simulink library "RobotX_Lib"  (R2026a)
settings: Solver=VariableStepAuto
settings Model: Creator=shueb  LastModifiedBy=shueb

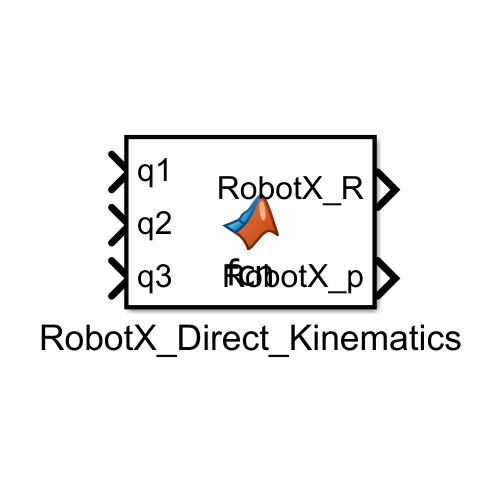
[thumbnail: Simulink's stored preview of the top-level diagram]
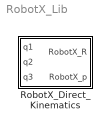
== system RobotX_Lib ==
  RobotX_Direct_Kinematics : MATLAB Function  TreatAsAtomicUnit=on

== matlab function RobotX_Lib/RobotX_Direct_Kinematics ==
  data: q1 input; RobotX_R output; q2 input; q3 input; RobotX_p output
function [RobotX_R,RobotX_p] = RobotX_Direct_Kinematics(q1,q2,q3)
%#codegen

%    This function was generated by the Symbolic Math Toolbox version 26.1.
%    24-Apr-2026 13:00:17

% q1 = complex(q1);  % if required to enforce complex operations
% q2 = complex(q2);  % if required to enforce complex operations
% q3 = complex(q3);  % if required to enforce complex operations
t2 = cos(q1);
t3 = cos(q2);
t4 = sin(q1);
t5 = sin(q2);
t6 = -t5;
RobotX_R = reshape([t2.*t6,t4.*t6,t3,t4,-t2,0.0,t2.*t3,t3.*t4,t5],[3,3]);
if nargout > 1
    t7 = q3.*t3.*2.0;
    t8 = t3+t6+t7;
    RobotX_p = [(t2.*t8)./2.0;(t4.*t8)./2.0;t3./2.0+t5./2.0+q3.*t5];
end
end
